simulink library "vmc"  (R2021b)
settings: Solver=VariableStepAuto  StartTime=0.0  StopTime=10.0  RelTol=1e-3
undefined symbols (not defined in the file or in its folder): AVMC_ACCDeltaTqIGain_X_kph, AVMC_ACCDeltaTqIGain_Y_mps2, AVMC_ACCDeltaTqPGain_X_kph, AVMC_ACCDeltaTqPGain_Y_kph, AVMC_ACCLongSteadyCtrl_X_kph, AVMC_AggressJerkPCT4AT_X_kph, AVMC_AggressJerkPCT_X_kph, AVMC_AggressLimitPCT4AT_X_kph, AVMC_AggressLimitPCT_X_kph, AVMC_CCLongSteadyCtrl_X_kph, AVMC_DISCDeltaTqIGain_X_kph, AVMC_DISCDeltaTqIGain_Y_mps2, AVMC_DISCDeltaTqPGain_X_kph, AVMC_DISCDeltaTqPGain_Y_kph, AVMC_DISCTrunAccJerk_X_s, AVMC_DISCTrunAccLimit_X_s, AVMC_ESCRegenOut_X_kph, AVMC_ESCRegenOut_Y_Deg, AVMC_ESCRegenOutEnSpd_X_Deg, AVMC_ISOAccLimit_X_mps, AVMC_ISODecLimit_X_mps, AVMC_ISOJerk_X_mps, AVMC_LatESCRegenOut_X_kph, AVMC_LatESCRegenOut_Y_Deg, AVMC_LongAccDeadZone_X_kph, AVMC_LongAccFiltTsforP2_X_Gps, AVMC_MCPresBaseTq_X_bar, AVMC_MSALongSteadyCtrl_X_kph, AVMC_MSAPedalOvrd2_X_kph, AVMC_MSAPedalOvrd_X_kph, AVMC_MSASpdBand_X_kph, AVMC_MSATqDownEndTq_X_kph, AVMC_MSATqDownTime_X_kph, AVMC_RDCDetectTime_X_kph, AVMC_RDCDetectTime_Y_pct, AVMC_RDCEnSlideRate_X_Deg, AVMC_RearWhlTqRatio_X_Nm, AVMC_RearWhlTqRatio_Y_gps, AVMC_RearWhlTqSlipGain_X_rat, AVMC_RearWhlTqSlipGain_Y_kph, AVMC_SoftJerkPCT_X_kph, AVMC_SoftLimitPCT_X_kph, AVMC_StESCYaw_X_kph, AVMC_StESCYaw_Y_Deg, AVMC_StESCYawCom_X_kph, AVMC_StESCYawCom_Y_Gps, AVMC_TMSpdBaseTq_X_rpm, AVMC_VehHoldBDecMap_X_kph, AVMC_VehHoldDecCtrlTime_X_kph, AVMC_VehHoldMCPPass_X_deg, C_TASK_10MS_S, C_TASK_5MS_S, DEG2RAD, Discrete, ENUM_ACCAVAIL_AVAILABLE, ENUM_ACCCTRLALLOW_ALLOW, ENUM_ADASACCSTA_ACTIVE, ENUM_ADASACCSTA_OVERRIDE, ENUM_ADASACCSTA_SHUTOFF, ENUM_ADASAEBREQ_NOREQUEST ... (+361)
libraries: hcu_lib x63, simulink x60, simulink_extras x3, ctrlSharedLib x3, $bdroot x2
(part 3 of 15)

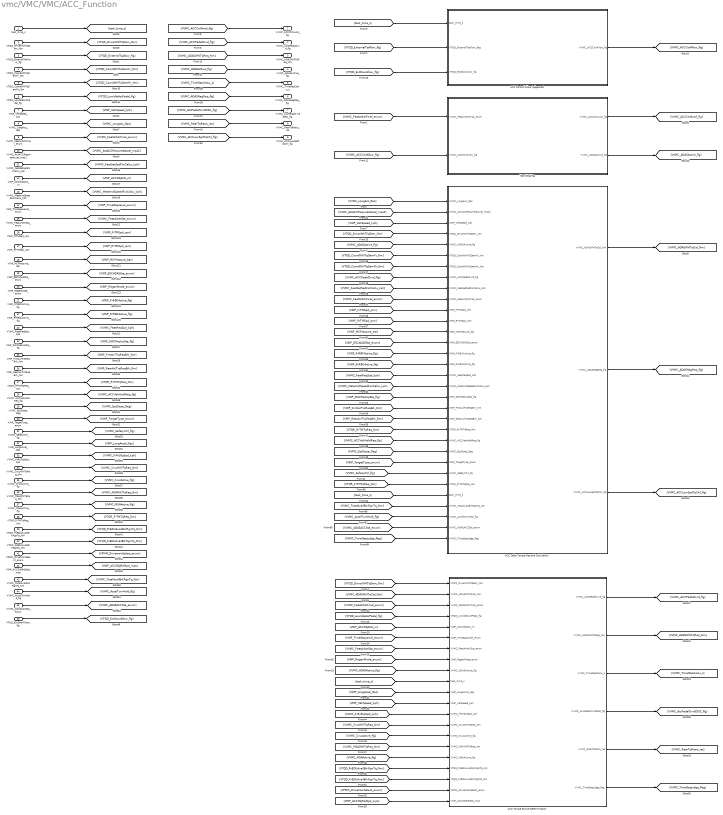
== system vmc/VMC/VMC/ACC_Function ==
  task_time_s : Inport
  VTQD_DriverWhlTqDem_Nm : Inport  Port=2
  VTQD_ExternalTqAllow_flg : Inport  Port=3
  VTQD_CoordWhlTqDemFr_Nm : Inport  Port=4
  VTQD_CoordWhlTqDemRr_Nm : Inport  Port=5
  VTQD_LowIdleAccPedal_flg : Inport  Port=6
  VINP_VehSpeed_kph : Inport  Port=7
  VVMC_LongAcc_Gps : Inport  Port=8
  VVMC_FeatArbitrFinal_enum : Inport  Port=9
  VVMC_ActACCRequiredAccel_mps2 : Inport  Port=10
  VVMC_FeatSetSpdForCalcu_kph : Inport  Port=11
  VINP_ACCObjDist_m : Inport  Port=12
  VVMC_MeterIndSpeedForCalcu_kph : Inport  Port=13
  VINP_TimeGapLevel_enum : Inport  Port=14
  VVMC_FeatArbitrSta_enum : Inport  Port=15
  VINP_FrTMSpd_rpm : Inport  Port=16
  VINP_RrTMSpd_rpm : Inport  Port=17
  VINP_MCPressure_bar : Inport  Port=18
  VINP_ESCADASSta_enum : Inport  Port=19
  VINP_RegenMode_enum : Inport  Port=20
  VINP_FrRBCActive_flg : Inport  Port=21
  VINP_RrRBCActive_flg : Inport  Port=22
  VVMC_FeatReqSpd_kph : Inport  Port=23
  VINP_SWCResUpSta_flg : Inport  Port=24
  VINP_FrntAxlTrqReqBrk_Nm : Inport  Port=25
  VINP_RearAxlTrqReqBrk_Nm : Inport  Port=26
  VTQR_RrTMTqReq_Nm : Inport  Port=27
  VVMC_ACCVehHoldReq_flg : Inport  Port=28
  VVMC_EstSlope_Deg : Inport  Port=29
  VINP_TargetType_enum : Inport  Port=30
  VVMC_SafetyCtrl_flg : Inport  Port=31
  VINP_LongAccel_Gps : Inport  Port=32
  VVMC_FrRrSlipSpd_kph : Inport  Port=33
  VVMC_CruzWhlTqReq_Nm : Inport  Port=34
  VVMC_CruzActive_flg : Inport  Port=35
  VVMC_MSAWhlTqReq_Nm : Inport  Port=36
  VVMC_MSAActive_flg : Inport  Port=37
  VTQR_FrTMTqReq_Nm : Inport  Port=38
  VTQD_RrEDUAvailBrkRgnTq_Nm : Inport  Port=39
  VTQD_FrEDUAvailBrkRgnTq_Nm : Inport  Port=40
  VPMM_DrivetrainSelect_enum : Inport  Port=41
  VINP_ACCObjRelSpd_mps : Inport  Port=42
  VVMC_TotalAvailBrkRgnTq_Nm : Inport  Port=43
  VVMC_AccelTurnHold_flg : Inport  Port=44
  VVMC_ADASACCSta_enum : Inport  Port=45
  VTQD_ExtDoorAllow_flg : Inport  Port=46
  ACC Control Allow Judgement : Subsystem
  ACC Delta Torque Map and Calculation : Subsystem
  ACC Torque Source Determination : Subsystem
  Hand Shaking : Subsystem
  VVMC_ACCCtrlAvail_flg : Outport
  VVMC_ACCPedalOvrd_flg : Outport  Port=2
  VVMC_ADASWhlTqReq_Nm : Outport  Port=3
  VVMC_ADASActive_flg : Outport  Port=4
  VVMC_TimeGapCalcu_s : Outport  Port=5
  VVMC_ADASNegReq_flg : Outport  Port=6
  VVMC_AccPedalOvrdDISC_flg : Outport  Port=7
  VVMC_RearTqRatio_rat : Outport  Port=8
  VVMC_ACCLowSpdTqCtrl_flg : Outport  Port=9
  wires:
  [VVMC_FeatReqSpd_kph] -> ACC Delta Torque Map and Calculation/17(VVMC_FeatReqSpd_kph)
  VVMC_FeatReqSpd_kph/1 -> [VVMC_FeatReqSpd_kph]
  [VVMC_ADASActive_flg] -> ACC Torque Source Determination/9(VVMC_ADASActive_flg)
  [VINP_RrRBCActive_flg] -> ACC Delta Torque Map and Calculation/16(VINP_RrRBCActive_flg)
  [VINP_FrRBCActive_flg] -> ACC Delta Torque Map and Calculation/15(VINP_FrRBCActive_flg)
  [VINP_ESCADASSta_enum] -> ACC Delta Torque Map and Calculation/14(VINP_ESCADASSta_enum)
  [VINP_MCPressure_bar] -> ACC Delta Torque Map and Calculation/13(VINP_MCPressure_bar)
  [VINP_RrTMSpd_rpm] -> ACC Delta Torque Map and Calculation/12(VINP_RrTMSpd_rpm)
  [VINP_FrTMSpd_rpm] -> ACC Delta Torque Map and Calculation/11(VINP_FrTMSpd_rpm)
  [VINP_RegenMode_enum] -> ACC Torque Source Determination/8(VINP_RegenMode_enum)
  VINP_FrTMSpd_rpm/1 -> [VINP_FrTMSpd_rpm]
  VINP_RrTMSpd_rpm/1 -> [VINP_RrTMSpd_rpm]
  VINP_MCPressure_bar/1 -> [VINP_MCPressure_bar]
  VINP_ESCADASSta_enum/1 -> [VINP_ESCADASSta_enum]
  VINP_RegenMode_enum/1 -> [VINP_RegenMode_enum]
  VINP_RrRBCActive_flg/1 -> [VINP_RrRBCActive_flg]
  VINP_FrRBCActive_flg/1 -> [VINP_FrRBCActive_flg]
  [VVMC_FeatArbitrFinal_enum] -> ACC Delta Torque Map and Calculation/10(VVMC_FeatArbitrFinal_enum)
  [VTQD_ExternalTqAllow_flg] -> ACC Control Allow Judgement/2(VTQD_ExternalTqAllow_flag)
  ACC Control Allow Judgement/1(VVMC_ACCCtrlAllow_flg) -> [VVMC_ACCCtrlAllow_flg]
  [task_time_s] -> ACC Control Allow Judgement/1(task_time_s)
  [VVMC_TimeGapCalcu_s] -> VVMC_TimeGapCalcu_s/1
  ACC Torque Source Determination/3(VVMC_TimeGapCalcu_s) -> [VVMC_TimeGapCalcu_s]
  [VVMC_FeatArbitrSta_enum] -> ACC Torque Source Determination/7(VVMC_FeatArbitrSta_enum)
  VVMC_FeatArbitrSta_enum/1 -> [VVMC_FeatArbitrSta_enum]
  [VINP_TimeGapLevel_enum] -> ACC Torque Source Determination/6(VINP_TimeGapLevel_enum)
  [VINP_ACCObjDist_m] -> ACC Torque Source Determination/5(VINP_ACCObjDist_m)
  VINP_TimeGapLevel_enum/1 -> [VINP_TimeGapLevel_enum]
  VINP_ACCObjDist_m/1 -> [VINP_ACCObjDist_m]
  VVMC_MeterIndSpeedForCalcu_kph/1 -> [VVMC_MeterIndSpeedForCalcu_kph]
  [VVMC_ACCPedalOvrd_flg] -> VVMC_ACCPedalOvrd_flg/1
  Hand Shaking/1(VVMC_ACCCtrlAvail_flg) -> [VVMC_ACCCtrlAvail_flg]
  VVMC_LongAcc_Gps/1 -> [VVMC_LongAcc_Gps]
  VVMC_FeatArbitrFinal_enum/1 -> [VVMC_FeatArbitrFinal_enum]
  VVMC_ActACCRequiredAccel_mps2/1 -> [VVMC_ActACCRequiredAccel_mps2]
  [VVMC_ACCCtrlAvail_flg] -> VVMC_ACCCtrlAvail_flg/1
  VTQD_ExternalTqAllow_flg/1 -> [VTQD_ExternalTqAllow_flg]
  VINP_VehSpeed_kph/1 -> [VINP_VehSpeed_kph]
  VTQD_DriverWhlTqDem_Nm/1 -> [VTQD_DriverWhlTqDem_Nm]
  [VVMC_LongAcc_Gps] -> ACC Delta Torque Map and Calculation/1(VVMC_LongAcc_Gps)
  [VVMC_ActACCRequiredAccel_mps2] -> ACC Delta Torque Map and Calculation/2(VVMC_ActACCRequiredAccel_mps2)
  [VINP_VehSpeed_kph] -> ACC Delta Torque Map and Calculation/3(VINP_VehSpeed_kph)
  [VTQD_DriverWhlTqDem_Nm] -> ACC Delta Torque Map and Calculation/4(VTQD_DriverWhlTqDem_Nm)
  ACC Delta Torque Map and Calculation/1(VVMC_ADASWhlTqCal_Nm) -> [VVMC_ADASWhlTqCal_Nm]
  [VTQD_DriverWhlTqDem_Nm] -> ACC Torque Source Determination/1(VTQD_DriverWhlTqDem_Nm)
  [VVMC_ADASWhlTqCal_Nm] -> ACC Torque Source Determination/2(VVMC_ADASWhlTqCal_Nm)
  ACC Torque Source Determination/1(VVMC_ACCPedalOvrd_flg) -> [VVMC_ACCPedalOvrd_flg]
  [VVMC_FeatArbitrFinal_enum] -> Hand Shaking/1(VVMC_FeatArbitrFinal_enum)
  Hand Shaking/2(VVMC_ADASActive_flg) -> [VVMC_ADASActive_flg]
  [VVMC_ADASActive_flg] -> ACC Delta Torque Map and Calculation/5(VVMC_ADASActive_flg)
  task_time_s/1 -> [task_time_s]
  [VVMC_ACCCtrlAllow_flg] -> Hand Shaking/2(VVMC_ACCCtrlAllow_flg)
  [VVMC_ADASActive_flg] -> VVMC_ADASActive_flg/1
  ACC Torque Source Determination/2(VVMC_ADASWhlTqReq_Nm) -> [VVMC_ADASWhlTqReq_Nm]
  [VVMC_ADASWhlTqReq_Nm] -> VVMC_ADASWhlTqReq_Nm/1
  [VTQD_CoordWhlTqDemFr_Nm] -> ACC Delta Torque Map and Calculation/6(VTQD_CoordWhlTqDemFr_Nm)
  [VTQD_CoordWhlTqDemRr_Nm] -> ACC Delta Torque Map and Calculation/7(VTQD_CoordWhlTqDemRr_Nm)
  VTQD_CoordWhlTqDemRr_Nm/1 -> [VTQD_CoordWhlTqDemRr_Nm]
  VTQD_CoordWhlTqDemFr_Nm/1 -> [VTQD_CoordWhlTqDemFr_Nm]
  [VVMC_ACCPedalOvrd_flg] -> ACC Delta Torque Map and Calculation/8(VVMC_ACCPedalOvrd_flg)
  [VVMC_FeatArbitrFinal_enum] -> ACC Torque Source Determination/3(VVMC_FeatArbitrFinal_enum)
  VTQD_LowIdleAccPedal_flg/1 -> [VTQD_LowIdleAccPedal_flg]
  [VTQD_LowIdleAccPedal_flg] -> ACC Torque Source Determination/4(VTQD_LowIdleAccPedal_flg)
  VVMC_FeatSetSpdForCalcu_kph/1 -> [VVMC_FeatSetSpdForCalcu_kph]
  [VVMC_FeatSetSpdForCalcu_kph] -> ACC Delta Torque Map and Calculation/9(VVMC_FeatSetSpdForCalcu_kph)
  VINP_SWCResUpSta_flg/1 -> [VINP_SWCResUpSta_flg]
  VINP_FrntAxlTrqReqBrk_Nm/1 -> [VINP_FrntAxlTrqReqBrk_Nm]
  VINP_RearAxlTrqReqBrk_Nm/1 -> [VINP_RearAxlTrqReqBrk_Nm]
  [VVMC_MeterIndSpeedForCalcu_kph] -> ACC Delta Torque Map and Calculation/18(VVMC_MeterIndSpeedForCalcu_kph)
  [VINP_SWCResUpSta_flg] -> ACC Delta Torque Map and Calculation/19(VINP_SWCResUpSta_flg)
  [VINP_FrntAxlTrqReqBrk_Nm] -> ACC Delta Torque Map and Calculation/20(VINP_FrntAxlTrqReqBrk_Nm)
  [VINP_RearAxlTrqReqBrk_Nm] -> ACC Delta Torque Map and Calculation/21(VINP_RearAxlTrqReqBrk_Nm)
  ACC Delta Torque Map and Calculation/2(VVMC_ADASNegReq_flg) -> [VVMC_ADASNegReq_flg]
  [VVMC_ADASNegReq_flg] -> VVMC_ADASNegReq_flg/1
  VTQR_RrTMTqReq_Nm/1 -> [VTQR_RrTMTqReq_Nm]
  [VTQR_RrTMTqReq_Nm] -> ACC Delta Torque Map and Calculation/22(VTQR_RrTMTqReq_Nm)
  ACC Torque Source Determination/4(VVMC_AccPedalOvrdDISC_flg) -> [VVMC_AccPedalOvrdDISC_flg]
  [VVMC_AccPedalOvrdDISC_flg] -> VVMC_AccPedalOvrdDISC_flg/1
  VVMC_ACCVehHoldReq_flg/1 -> [VVMC_ACCVehHoldReq_flg]
  [VVMC_ACCVehHoldReq_flg] -> ACC Delta Torque Map and Calculation/23(VVMC_ACCVehHoldReq_flg)
  VVMC_EstSlope_Deg/1 -> [VVMC_EstSlope_Deg]
  [VVMC_EstSlope_Deg] -> ACC Delta Torque Map and Calculation/24(VVMC_EstSlope_Deg)
  [VINP_TargetType_enum] -> ACC Delta Torque Map and Calculation/25(VINP_TargetType_enum)
  VINP_TargetType_enum/1 -> [VINP_TargetType_enum]
  [task_time_s] -> ACC Torque Source Determination/10(task_time_s)
  VVMC_SafetyCtrl_flg/1 -> [VVMC_SafetyCtrl_flg]
  [VVMC_SafetyCtrl_flg] -> ACC Delta Torque Map and Calculation/26(VVMC_SafetyCtrl_flg)
  [VINP_LongAccel_Gps] -> ACC Torque Source Determination/11(VINP_LongAccel_Gps)
  ACC Torque Source Determination/5(VVMC_RearTqRatio_rat) -> [VVMC_RearTqRatio_rat]
  [VVMC_RearTqRatio_rat] -> VVMC_RearTqRatio_rat/1
  VINP_LongAccel_Gps/1 -> [VINP_LongAccel_Gps]
  VVMC_FrRrSlipSpd_kph/1 -> [VVMC_FrRrSlipSpd_kph]
  [VINP_VehSpeed_kph] -> ACC Torque Source Determination/12(VINP_VehSpeed_kph)
  [VVMC_FrRrSlipSpd_kph] -> ACC Torque Source Determination/13(VVMC_FrRrSlipSpd_kph)
  VVMC_MSAActive_flg/1 -> [VVMC_MSAActive_flg]
  VVMC_MSAWhlTqReq_Nm/1 -> [VVMC_MSAWhlTqReq_Nm]
  VVMC_CruzActive_flg/1 -> [VVMC_CruzActive_flg]
  VVMC_CruzWhlTqReq_Nm/1 -> [VVMC_CruzWhlTqReq_Nm]
  [VVMC_CruzWhlTqReq_Nm] -> ACC Torque Source Determination/14(VVMC_CruzWhlTqReq_Nm)
  [VVMC_CruzActive_flg] -> ACC Torque Source Determination/15(VVMC_CruzActive_flg)
  [VVMC_MSAWhlTqReq_Nm] -> ACC Torque Source Determination/16(VVMC_MSAWhlTqReq_Nm)
  [VVMC_MSAActive_flg] -> ACC Torque Source Determination/17(VVMC_MSAActive_flg)
  [VTQR_FrTMTqReq_Nm] -> ACC Delta Torque Map and Calculation/27(VTQR_FrTMTqReq_Nm)
  VTQR_FrTMTqReq_Nm/1 -> [VTQR_FrTMTqReq_Nm]
  VTQD_RrEDUAvailBrkRgnTq_Nm/1 -> [VTQD_RrEDUAvailBrkRgnTq_Nm]
  VTQD_FrEDUAvailBrkRgnTq_Nm/1 -> [VTQD_FrEDUAvailBrkRgnTq_Nm]
  [VTQD_RrEDUAvailBrkRgnTq_Nm] -> ACC Torque Source Determination/18(VTQD_RrEDUAvailBrkRgnTq_Nm)
  [VTQD_FrEDUAvailBrkRgnTq_Nm] -> ACC Torque Source Determination/19(VTQD_FrEDUAvailBrkRgnTq_Nm)
  ACC Delta Torque Map and Calculation/3(VVMC_ACCLowSpdTqCtrl_flg) -> [VVMC_ACCLowSpdTqCtrl_flg]
  [VVMC_ACCLowSpdTqCtrl_flg] -> VVMC_ACCLowSpdTqCtrl_flg/1
  VPMM_DrivetrainSelect_enum/1 -> [VPMM_DrivetrainSelect_enum]
  [VPMM_DrivetrainSelect_enum] -> ACC Torque Source Determination/20(VPMM_DrivetrainSelect_enum)
  [task_time_s] -> ACC Delta Torque Map and Calculation/28(task_time_s)
  VINP_ACCObjRelSpd_mps/1 -> [VINP_ACCObjRelSpd_mps]
  [VINP_ACCObjRelSpd_mps] -> ACC Torque Source Determination/21(VINP_ACCObjRelSpd_mps)
  VVMC_TotalAvailBrkRgnTq_Nm/1 -> [VVMC_TotalAvailBrkRgnTq_Nm]
  [VVMC_TotalAvailBrkRgnTq_Nm] -> ACC Delta Torque Map and Calculation/29(VVMC_TotalAvailBrkRgnTq_Nm)
  VVMC_AccelTurnHold_flg/1 -> [VVMC_AccelTurnHold_flg]
  [VVMC_AccelTurnHold_flg] -> ACC Delta Torque Map and Calculation/30(VVMC_AccelTurnHold_flg)
  VVMC_ADASACCSta_enum/1 -> [VVMC_ADASACCSta_enum]
  [VVMC_ADASACCSta_enum] -> ACC Delta Torque Map and Calculation/31(VVMC_ADASACCSta_enum)
  ACC Torque Source Determination/6(VVMC_TimeGapJudge_flag) -> [VVMC_TimeGapJudge_flag]
  [VVMC_TimeGapJudge_flag] -> ACC Delta Torque Map and Calculation/32(VVMC_TimeGapJudge_flag)
  [VTQD_ExtDoorAllow_flg] -> ACC Control Allow Judgement/3(VTQD_ExtDoorAllow_flg)
  VTQD_ExtDoorAllow_flg/1 -> [VTQD_ExtDoorAllow_flg]

== system vmc/VMC/VMC/APS function ==
  VTQD_ExternalTqAllow_flg : Inport
  VTQD_ExtShiftAllow_flg : Inport  Port=2
  VTQD_ExtDoorAllow_flg : Inport  Port=3
  VTQD_GearActualPosn_enum : Inport  Port=4
  VINP_APSStaSys_enum : Inport  Port=5
  VINP_APSVMCReqA_flg : Inport  Port=6
  VINP_APSShiftPosnReq_enum : Inport  Port=7
  VINP_APSSpeedCMD_kph : Inport  Port=8
  task_time_s : Inport  Port=9
  VINP_SCPSystemMode_enum : Inport  Port=10
  VVMC_ADASActive_flg : Inport  Port=11
  BINP_APM_outputs : Inport  Port=12  OutDataTypeStr=Bus: BINP_APM_outputs
  VTQD_APSStaSys_enum : Inport  Port=13
  VTQD_APSDecReqA_flg : Inport  Port=14
  VTQD_APSDecReq_mps2 : Inport  Port=15
  VTQD_APSReq_enum : Inport  Port=16
  Command Determination : Subsystem
  Data Type Conversion : DataTypeConversion  OutDataTypeStr=uint8
  Hand Shake : Subsystem
  Signal Rounting : Subsystem
  VVMC_APSCtrlAvail_flg : Outport
  VVMC_APSActive_flg : Outport  Port=2
  VVMC_APSSpeedCMD_kph : Outport  Port=3
  VVMC_APSShiftPosnReq_enum : Outport  Port=4
  VVMC_APSStaSys_enum : Outport  Port=5
  VVMC_APSDecReqA_flg : Outport  Port=6
  VVMC_APSDecReq_mps2 : Outport  Port=7
  VVMC_APSReq_enum : Outport  Port=8
  wires:
  Command Determination/2(VVMC_APSShiftPosnReq_enum) -> VVMC_APSShiftPosnReq_enum/1
  Command Determination/1(VVMC_APSSpeedCMD_kph) -> VVMC_APSSpeedCMD_kph/1
  [VINP_APSSpeedCMD_kph] -> Command Determination/4(VINP_APSSpeedCMD_kph)
  [VINP_APSShiftPosnReq_enum] -> Command Determination/3(VINP_APSShiftPosnReq_enum)
  [VINP_APSStaSys_enum] -> Command Determination/2(VINP_APSStaSys_enum)
  [VVMC_APSActive_flg] -> Command Determination/1(VVMC_APSActive_flg)
  Hand Shake/1(VVMC_APSCtrlAvail_flg) -> VVMC_APSCtrlAvail_flg/1
  Hand Shake/2(VVMC_APSActive_flg) -> VVMC_APSActive_flg/1, [VVMC_APSActive_flg]
  [VTQD_ExtShiftAllow_flg] -> Hand Shake/3(VTQD_ExtShiftAllow_flg)
  [VTQD_ExternalTqAllow_flg] -> Hand Shake/2(VTQD_ExternalTqAllow_flg)
  [task_time_s] -> Hand Shake/1(task_time_s)
  task_time_s/1 -> [task_time_s]
  VINP_APSSpeedCMD_kph/1 -> [VINP_APSSpeedCMD_kph]
  VINP_APSShiftPosnReq_enum/1 -> [VINP_APSShiftPosnReq_enum]
  VINP_APSVMCReqA_flg/1 -> [VINP_APSVMCReqA_flg]
  VINP_APSStaSys_enum/1 -> [VINP_APSStaSys_enum]
  VVMC_ADASActive_flg/1 -> [VVMC_ADASActive_flg]
  [VVMC_APSActive_flg] -> Signal Rounting/2(VVMC_APSActive_flg)
  [VVMC_ADASActive_flg] -> Signal Rounting/3(VVMC_ADASActive_flg)
  Signal Rounting/1(VVMC_APSStaSys_enum) -> VVMC_APSStaSys_enum/1
  Signal Rounting/4(VVMC_APSReq_enum) -> VVMC_APSReq_enum/1
  Signal Rounting/3(VVMC_APSDecReq_mps2) -> VVMC_APSDecReq_mps2/1
  Signal Rounting/2(VVMC_APSDecReqA_flg) -> VVMC_APSDecReqA_flg/1
  VTQD_ExtDoorAllow_flg/1 -> [VTQD_ExtDoorAllow_flg]
  VTQD_ExternalTqAllow_flg/1 -> [VTQD_ExternalTqAllow_flg]
  VTQD_ExtShiftAllow_flg/1 -> [VTQD_ExtShiftAllow_flg]
  VINP_SCPSystemMode_enum/1 -> Data Type Conversion/1
  [VTQD_ExtDoorAllow_flg] -> Hand Shake/6(VTQD_ExtDoorAllow_flg)
  [BINP_APM_outputs] -> Signal Rounting/4(BINP_APM_outputs)
  [VINP_APSVMCReqA_flg] -> Hand Shake/4(VINP_APSVMCReqA_flg)
  [VINP_APSStaSys_enum] -> Hand Shake/5(VINP_APSStaSys_enum)
  BINP_APM_outputs/1 -> [BINP_APM_outputs]
  VTQD_GearActualPosn_enum/1 -> [VTQD_GearActualPosn_enum]
  [VINP_SCPSystemMode_enum] -> Signal Rounting/1(VINP_SCPSystemMode_enum)
  [VTQD_GearActualPosn_enum] -> Signal Rounting/5(VTQD_GearActualPosn_enum)
  Data Type Conversion/1 -> [VINP_SCPSystemMode_enum]
  VTQD_APSStaSys_enum/1 -> [VTQD_APSStaSys_enum]
  VTQD_APSDecReq_mps2/1 -> [VTQD_APSDecReq_mps2]
  VTQD_APSDecReqA_flg/1 -> [VTQD_APSDecReqA_flg]
  VTQD_APSReq_enum/1 -> [VTQD_APSReq_enum]
  [VTQD_APSStaSys_enum] -> Signal Rounting/6(VTQD_APSStaSys_enum)
  [VTQD_APSDecReqA_flg] -> Signal Rounting/7(VTQD_APSDecReqA_flg)
  [VTQD_APSDecReq_mps2] -> Signal Rounting/8(VTQD_APSDecReq_mps2)
  [VTQD_APSReq_enum] -> Signal Rounting/9(VTQD_APSReq_enum)

== system vmc/VMC/VMC/CruiseControlFunction ==
  VTQD_ExternalTqAllow_flg : Inport
  VTQD_DriverWhlTqDem_Nm : Inport  Port=2
  VTQD_LowIdleAccPedal_flg : Inport  Port=3
  <VINP_ZoneSpdCtrlMode_enum> : Inport  Port=4
  VINP_SWCResUpSta_flg : Inport  Port=5
  VINP_SWCSetdownSta_flg : Inport  Port=6
  VINP_SWCCANCELSta_flg : Inport  Port=7
  VINP_BrakeSWGPIO_flg : Inport  Port=8
  VINP_BrkSwSta_flg : Inport  Port=9
  VINP_VehSpeed_kph : Inport  Port=10
  VVMC_LongAcc_Gps : Inport  Port=11
  VVMC_FeatSetSpdForCalcu_kph : Inport  Port=12
  VVMC_FeatArbitrFinal_enum : Inport  Port=13
  VINP_ADASAEBSta_enum : Inport  Port=14
  VTQD_GearActualPosn_enum : Inport  Port=15
  VVMC_CalMeterSpeed_kph : Inport  Port=16
  VVMC_MeterIndSpeedForCalcu_kph : Inport  Port=17
  VVMC_SafetyCtrl_flg : Inport  Port=18
  VTQR_FrTMTqReq_Nm : Inport  Port=19
  VTQR_RrTMTqReq_Nm : Inport  Port=20
  VINP_RegenMode_enum : Inport  Port=21
  VVMC_ActACCRequiredAccel_mps2 : Inport  Port=22
  task_time_s : Inport  Port=23
  VVMC_TotalAvailBrkRgnTq_Nm : Inport  Port=24
  CCActiveDetermination : Subsystem
  CCDemandTorqueCalculation : Subsystem
  CCTorqueSourceDetermination : Subsystem
  Data Type Conversion : DataTypeConversion  OutDataTypeStr=single
  VVMC_CCCtrlSta_enum : Outport
  VVMC_CCSpdWar_flg : Outport  Port=2
  VVMC_CruzWhlTqReq_Nm : Outport  Port=3
  VVMC_CruzActive_flg : Outport  Port=4
  VVMC_CCPedalOvrd_flg : Outport  Port=5
  wires:
  [VVMC_CCPedalOvrd_flg] -> VVMC_CCPedalOvrd_flg/1
  [VVMC_CCPedalOvrd_flg] -> CCActiveDetermination/12(VVMC_CCPedalOvrd_flg)
  [VINP_ADASAEBSta_enum] -> CCActiveDetermination/11(VINP_ADASAEBSta_enum)
  VINP_ADASAEBSta_enum/1 -> [VINP_ADASAEBSta_enum]
  [VINP_ZoneSpdCtrlMode_enum] -> CCActiveDetermination/1(VINP_ZoneSpdCtrlMode_enum)
  <VINP_ZoneSpdCtrlMode_enum>/1 -> [VINP_ZoneSpdCtrlMode_enum]
  [VVMC_FeatArbitrFinal_enum] -> CCActiveDetermination/2(VVMC_FeatArbitrFinal_enum)
  [VTQD_ExternalTqAllow_flg] -> CCActiveDetermination/3(VTQD_ExternalTqAllow_flg)
  [VINP_SWCSetdownSta_flg] -> CCActiveDetermination/4(VINP_SWCSetdownSta_flg)
  [VINP_SWCResUpSta_flg] -> CCActiveDetermination/5(VINP_SWCResUpSta_flg)
  [VVMC_FeatSetSpdForCalcu_kph] -> CCActiveDetermination/7(VVMC_FeatSetSpdForCalcu_kph)
  [VINP_BrakeSWGPIO_flg] -> CCActiveDetermination/8(VINP_BrakeSWGPIO_flg)
  [VINP_SWCCANCELSta_flg] -> CCActiveDetermination/9(VINP_SWCCANCELSta_flg)
  [VINP_BrkSwSta_flg] -> CCActiveDetermination/10(VINP_BrkSwSta_flg)
  [VVMC_FeatSetSpdForCalcu_kph] -> CCDemandTorqueCalculation/1(VVMC_FeatSetSpdForCalcu_kph)
  [VINP_VehSpeed_kph] -> CCDemandTorqueCalculation/2(VINP_VehSpeed_kph)
  [VVMC_CruzActive_flg] -> CCDemandTorqueCalculation/3(VVMC_CruzActive_flg)
  [VTQD_DriverWhlTqDem_Nm] -> CCDemandTorqueCalculation/4(VTQD_DriverWhlTqDem_Nm)
  [VTQD_DriverWhlTqDem_Nm] -> CCTorqueSourceDetermination/1(VTQD_DriverWhlTqDem_Nm)
  [VVMC_CruzWhlTqCal_Nm] -> CCTorqueSourceDetermination/2(VVMC_CruzWhlTqCal_Nm)
  CCActiveDetermination/1(VVMC_CCCtrlSta_enum) -> [VVMC_CCCtrlSta_enum]
  CCActiveDetermination/2(VVMC_CCSpdWar_flg) -> [VVMC_CCSpdWar_flg]
  CCActiveDetermination/3(VVMC_CruzActive_flg) -> [VVMC_CruzActive_flg]
  CCDemandTorqueCalculation/1(VVMC_CruzWhlTqCal_Nm) -> [VVMC_CruzWhlTqCal_Nm]
  CCTorqueSourceDetermination/1(VVMC_CruzWhlTqReq_Nm) -> [VVMC_CruzWhlTqReq_Nm]  "VVMC_CruzWhlTqReq_Nm"
  VTQD_ExternalTqAllow_flg/1 -> [VTQD_ExternalTqAllow_flg]
  VTQD_DriverWhlTqDem_Nm/1 -> [VTQD_DriverWhlTqDem_Nm]
  VINP_SWCResUpSta_flg/1 -> [VINP_SWCResUpSta_flg]
  VINP_SWCSetdownSta_flg/1 -> [VINP_SWCSetdownSta_flg]
  VINP_SWCCANCELSta_flg/1 -> [VINP_SWCCANCELSta_flg]
  VINP_BrakeSWGPIO_flg/1 -> [VINP_BrakeSWGPIO_flg]
  VVMC_FeatSetSpdForCalcu_kph/1 -> Data Type Conversion/1
  VINP_BrkSwSta_flg/1 -> [VINP_BrkSwSta_flg]
  VVMC_FeatArbitrFinal_enum/1 -> [VVMC_FeatArbitrFinal_enum]
  VINP_VehSpeed_kph/1 -> [VINP_VehSpeed_kph]
  [VVMC_CCCtrlSta_enum] -> VVMC_CCCtrlSta_enum/1
  [VVMC_CCSpdWar_flg] -> VVMC_CCSpdWar_flg/1
  [VVMC_CruzWhlTqReq_Nm] -> VVMC_CruzWhlTqReq_Nm/1
  Data Type Conversion/1 -> [VVMC_FeatSetSpdForCalcu_kph]  "VVMC_FeatSetSpdForCalcu_kph"
  [VVMC_CruzActive_flg] -> VVMC_CruzActive_flg/1
  VVMC_LongAcc_Gps/1 -> [VVMC_LongAcc_Gps]
  [VVMC_LongAcc_Gps] -> CCDemandTorqueCalculation/5(VVMC_LongAcc_Gps)
  [VINP_VehSpeed_kph] -> CCActiveDetermination/6(VINP_VehSpeed_kph)
  VTQD_LowIdleAccPedal_flg/1 -> [VTQD_LowIdleAccPedal_flg]
  [VTQD_LowIdleAccPedal_flg] -> CCTorqueSourceDetermination/3(VTQD_LowIdleAccPedal_flg)
  CCTorqueSourceDetermination/2(VVMC_CCPedalOvrd_flg) -> [VVMC_CCPedalOvrd_flg]  "VVMC_CCPedalOvrd_flg"
  [VVMC_CCPedalOvrd_flg] -> CCDemandTorqueCalculation/6(VVMC_CCPedalOvrd_flg)
  VTQD_GearActualPosn_enum/1 -> [VTQD_GearActualPosn_enum]
  [VTQD_GearActualPosn_enum] -> CCActiveDetermination/13(VTQD_GearActualPosn_enum)
  VVMC_CalMeterSpeed_kph/1 -> [VVMC_CalMeterSpeed_kph]
  [VVMC_CalMeterSpeed_kph] -> CCDemandTorqueCalculation/7(VVMC_CalMeterSpeed_kph)
  [VVMC_FeatArbitrFinal_enum] -> CCDemandTorqueCalculation/8(VVMC_FeatArbitrFinal_enum)
  [VVMC_MeterIndSpeedForCalcu_kph] -> CCDemandTorqueCalculation/10(VVMC_MeterIndSpeedForCalcu_kph)
  VVMC_MeterIndSpeedForCalcu_kph/1 -> [VVMC_MeterIndSpeedForCalcu_kph]
  [VVMC_SafetyCtrl_flg] -> CCDemandTorqueCalculation/11(VVMC_SafetyCtrl_flg)
  VVMC_SafetyCtrl_flg/1 -> [VVMC_SafetyCtrl_flg]
  [VTQR_FrTMTqReq_Nm] -> CCDemandTorqueCalculation/12(VTQR_FrTMTqReq_Nm)
  [VTQR_RrTMTqReq_Nm] -> CCDemandTorqueCalculation/13(VTQR_RrTMTqReq_Nm)
  VTQR_FrTMTqReq_Nm/1 -> [VTQR_FrTMTqReq_Nm]
  VTQR_RrTMTqReq_Nm/1 -> [VTQR_RrTMTqReq_Nm]
  [VINP_RegenMode_enum] -> CCTorqueSourceDetermination/4(VINP_RegenMode_enum)
  [VVMC_FeatArbitrFinal_enum] -> CCTorqueSourceDetermination/5(VVMC_FeatArbitrFinal_enum)
  VINP_RegenMode_enum/1 -> [VINP_RegenMode_enum]
  [task_time_s] -> CCTorqueSourceDetermination/6(task_time_s)
  VVMC_ActACCRequiredAccel_mps2/1 -> [VVMC_ActACCRequiredAccel_mps2]
  task_time_s/1 -> [task_time_s]
  [VVMC_ActACCRequiredAccel_mps2] -> CCDemandTorqueCalculation/9(VVMC_ActACCRequiredAccel_mps2)
  VVMC_TotalAvailBrkRgnTq_Nm/1 -> [VVMC_TotalAvailBrkRgnTq_Nm]
  [VVMC_TotalAvailBrkRgnTq_Nm] -> CCDemandTorqueCalculation/14(VVMC_TotalAvailBrkRgnTq_Nm)

== system vmc/VMC/VMC/FeatureSetSpeed ==
  APP_SpdLimit_flg : Inport
  VINP_ZoneSpdCtrlSta_flg : Inport  Port=2
  APP_SpdLimit : Inport  Port=3
  VINP_SetSpd_kph : Inport  Port=4
  VINP_Distanceunit_flg : Inport  Port=5
  Cast To Single : DataTypeConversion  OutDataTypeStr=single
  Cast To Single1 : DataTypeConversion  OutDataTypeStr=single
  Constant : Constant  Value=ENUM_SCPCRLSTA_ON
  Constant1 : Constant  Value=ENUM_APPSPDLIMIT_ON
  Constant2 : Constant  Value=ZERO_FLOAT
  Constant4 : Constant  Value=MPH2KPH
  Constant5 : Constant  Value=KVMC_APPSpdLimit_flg_ovrdflg
  Constant6 : Constant  Value=KVMC_APPSpdLimit_flg_ovrdval
  Constant7 : Constant  Value=KVMC_APPSpdLimit_ovrdflg
  Constant8 : Constant  Value=KVMC_APPSpdLimit_ovrdval
  Divide1 : Product  Inputs=**
  Round1 : Rounding  Operator=ceil
  SpeedDetermination : Stateflow chart  TreatAsAtomicUnit=on
  Switch : Switch  Criteria=u2 ~= 0
  Switch1 : Switch  Criteria=u2 ~= 0
  u2 > 0 (2) : Switch  Criteria=u2 > Threshold
  VVMC_FeatSetSpdFinal_raw32 : Outport
  VVMC_FeatSetSpdForCalcu_kph : Outport  Port=2
  wires:
  [VINP_SetSpd_kph] -> SpeedDetermination/4(VINP_SetSpd_kph)
  Constant2/1 -> SpeedDetermination/7(ZERO_FLOAT)
  Constant6/1 -> Switch/1
  Constant1/1 -> SpeedDetermination/6(ENUM_APPSPDLIMIT_ON)
  Constant5/1 -> Switch/2
  [APP_SpdLimit_flg] -> Switch/3
  SpeedDetermination/1(VVMC_FeatSetSpdFinal_raw32) -> Cast To Single/1
  Constant/1 -> SpeedDetermination/5(ENUM_SCPCRLSTA_ON)
  Switch1/1 -> [VVMC_APPSpdLimit_kph]  "VVMC_APPSpdLimit_kph"
  Constant8/1 -> Switch1/1
  [APP_SpdLimit] -> Switch1/3
  [VINP_ZoneSpdCtrlSta_flg] -> SpeedDetermination/2(VINP_ZoneSpdCtrlSta_flg)
  Constant7/1 -> Switch1/2
  [VVMC_APPSpdLimit_flg] -> SpeedDetermination/1(VVMC_APPSpdLimit_flg)
  Switch/1 -> [VVMC_APPSpdLimit_flg]  "VVMC_APPSpdLimit_flg"
  Cast To Single/1 -> [VVMC_FeatSetSpdFinal_raw32]  "VVMC_FeatSetSpdFinal_raw32"
  [VVMC_APPSpdLimit_kph] -> SpeedDetermination/3(VVMC_APPSpdLimit_kph)
  APP_SpdLimit_flg/1 -> [APP_SpdLimit_flg]
  VINP_ZoneSpdCtrlSta_flg/1 -> [VINP_ZoneSpdCtrlSta_flg]
  APP_SpdLimit/1 -> [APP_SpdLimit]
  VINP_SetSpd_kph/1 -> [VINP_SetSpd_kph]
  [VVMC_FeatSetSpdFinal_raw32] -> VVMC_FeatSetSpdFinal_raw32/1
  [VVMC_FeatSetSpdFinal_raw32] -> Divide1/1, u2 > 0 (2)/3
  u2 > 0 (2)/1 -> Cast To Single1/1
  Constant4/1 -> Divide1/2
  Divide1/1 -> u2 > 0 (2)/1
  [VINP_Distanceunit_flg] -> u2 > 0 (2)/2
  Round1/1 -> [VVMC_FeatSetSpdForCalcu_kph]  "VVMC_FeatSetSpdForCalcu_kph"
  Cast To Single1/1 -> Round1/1
  [VVMC_FeatSetSpdForCalcu_kph] -> VVMC_FeatSetSpdForCalcu_kph/1
  VINP_Distanceunit_flg/1 -> [VINP_Distanceunit_flg]

== system vmc/VMC/VMC/IMU ==
  VINP_MemOffsetGyroX_raw16 : Inport
  VINP_MemOffsetGyroY_raw16 : Inport  Port=2
  VINP_MemOffsetGyroZ_raw16 : Inport  Port=3
  VINP_MemOffsetAccX_raw16 : Inport  Port=4
  VINP_MemOffsetAccY_raw16 : Inport  Port=5
  VINP_MemOffsetAccZ_raw16 : Inport  Port=6
  VINP_SensingGyroX_raw16 : Inport  Port=7
  VINP_SensingGyroY_raw16 : Inport  Port=8
  VINP_SensingGyroZ_raw16 : Inport  Port=9
  VINP_SensingAccX_raw16 : Inport  Port=10
  VINP_SensingAccY_raw16 : Inport  Port=11
  VINP_SensingAccZ_raw16 : Inport  Port=12
  task_time_s : Inport  Port=13
  Constant : Constant  Value=KVMC_IMUEnaCmd_flg
  IMU memorized offset result : Subsystem
  "IMU sensing result " : Subsystem
  VVMC_IMUEnaCmd_flg : Outport
  wires:
  VINP_MemOffsetGyroX_raw16/1 -> [VINP_MemOffsetGyroX_raw16]
  VINP_MemOffsetGyroY_raw16/1 -> [VINP_MemOffsetGyroY_raw16]
  VINP_MemOffsetGyroZ_raw16/1 -> [VINP_MemOffsetGyroZ_raw16]
  VINP_MemOffsetAccX_raw16/1 -> [VINP_MemOffsetAccX_raw16]
  VINP_MemOffsetAccY_raw16/1 -> [VINP_MemOffsetAccY_raw16]
  VINP_MemOffsetAccZ_raw16/1 -> [VINP_MemOffsetAccZ_raw16]
  VINP_SensingGyroX_raw16/1 -> [VINP_SensingGyroX_raw16]
  VINP_SensingGyroY_raw16/1 -> [VINP_SensingGyroY_raw16]
  VINP_SensingGyroZ_raw16/1 -> [VINP_SensingGyroZ_raw16]
  VINP_SensingAccX_raw16/1 -> [VINP_SensingAccX_raw16]
  VINP_SensingAccY_raw16/1 -> [VINP_SensingAccY_raw16]
  VINP_SensingAccZ_raw16/1 -> [VINP_SensingAccZ_raw16]
  [VINP_MemOffsetGyroX_raw16] -> IMU memorized offset result/1(VINP_MemOffsetGyroX_raw16)
  [VINP_MemOffsetGyroY_raw16] -> IMU memorized offset result/2(VINP_MemOffsetGyroY_raw16)
  [VINP_MemOffsetGyroZ_raw16] -> IMU memorized offset result/3(VINP_MemOffsetGyroZ_raw16)
  [VINP_MemOffsetAccX_raw16] -> IMU memorized offset result/4(VINP_MemOffsetAccX_raw16)
  [VINP_MemOffsetAccY_raw16] -> IMU memorized offset result/5(VINP_MemOffsetAccY_raw16)
  [VINP_MemOffsetAccZ_raw16] -> IMU memorized offset result/6(VINP_MemOffsetAccZ_raw16)
  IMU memorized offset result/6(VVMC_MemOffsetAccZ_G) -> [VVMC_MemOffsetAccZ_G]
  IMU memorized offset result/5(VVMC_MemOffsetAccY_G) -> [VVMC_MemOffsetAccY_G]
  IMU memorized offset result/4(VVMC_MemOffsetAccX_G) -> [VVMC_MemOffsetAccX_G]
  IMU memorized offset result/3(VVMC_MemOffsetGyroZ_Dps) -> [VVMC_MemOffsetGyroZ_Dps]
  IMU memorized offset result/2(VVMC_MemOffsetGyroY_Dps) -> [VVMC_MemOffsetGyroY_Dps]
  IMU memorized offset result/1(VVMC_MemOffsetGyroX_Dps) -> [VVMC_MemOffsetGyroX_Dps]
  [VVMC_MemOffsetGyroY_Dps] -> "IMU sensing result "/8(VVMC_MemOffsetGyroY_Dps)
  [VVMC_MemOffsetAccX_G] -> "IMU sensing result "/10(VVMC_MemOffsetAccX_G)
  [VVMC_MemOffsetGyroZ_Dps] -> "IMU sensing result "/9(VVMC_MemOffsetGyroZ_Dps)
  [VVMC_MemOffsetAccY_G] -> "IMU sensing result "/11(VVMC_MemOffsetAccY_G)
  [VVMC_MemOffsetGyroX_Dps] -> "IMU sensing result "/7(VVMC_MemOffsetGyroX_Dps)
  [VVMC_MemOffsetAccZ_G] -> "IMU sensing result "/12(VVMC_MemOffsetAccZ_G)
  [VINP_SensingGyroX_raw16] -> "IMU sensing result "/1(VINP_SensingGyroX_raw16)
  [VINP_SensingAccZ_raw16] -> "IMU sensing result "/6(VINP_SensingAccZ_raw16)
  [VINP_SensingAccY_raw16] -> "IMU sensing result "/5(VINP_SensingAccY_raw16)
  [VINP_SensingAccX_raw16] -> "IMU sensing result "/4(VINP_SensingAccX_raw16)
  [VINP_SensingGyroZ_raw16] -> "IMU sensing result "/3(VINP_SensingGyroZ_raw16)
  [VINP_SensingGyroY_raw16] -> "IMU sensing result "/2(VINP_SensingGyroY_raw16)
  Constant/1 -> [VVMC_IMUEnaCmd_flg]  "VVMC_IMUEnaCmd_flg"
  [VVMC_IMUEnaCmd_flg] -> VVMC_IMUEnaCmd_flg/1
  task_time_s/1 -> [task_time_s]
  [task_time_s] -> "IMU sensing result "/13(task_time_s)

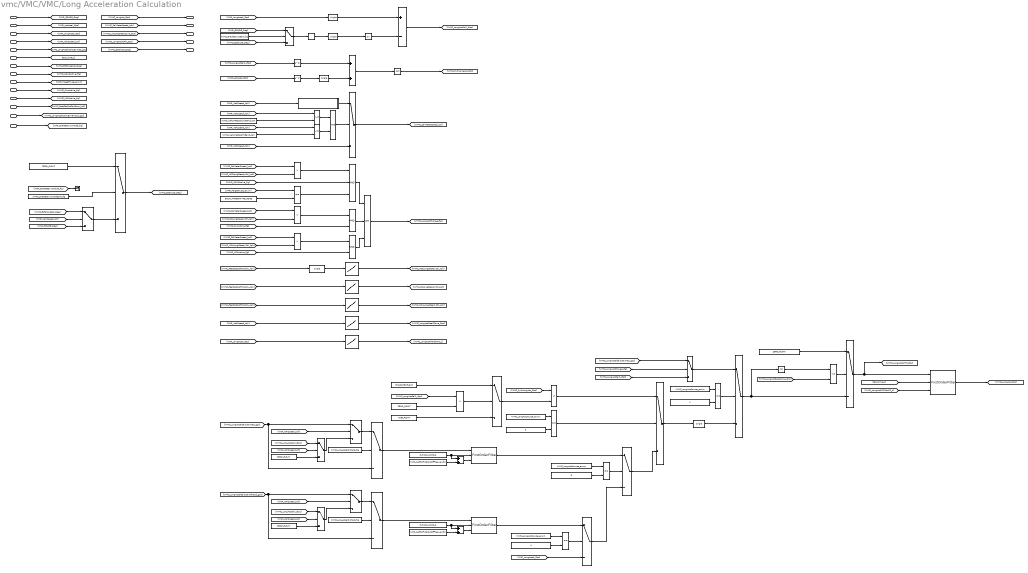
== system vmc/VMC/VMC/Long Acceleration Calculation ==
  VINP_GRADE_Deg : Inport
  VINP_LatAccel_Gps : Inport  Port=2
  VINP_LongAccel_Gps : Inport  Port=3
  VINP_VehSpeed_kph : Inport  Port=4
  VVMC_LongAccelCalcuByWSS_gps : Inport  Port=5
  task_time_s : Inport  Port=6
  VVMC_EstSlopeCal_Deg : Inport  Port=7
  VVMC_ADASActive_flg : Inport  Port=8
  VINP_TargetType_enum : Inport  Port=9
  VVMC_CruzActive_flg : Inport  Port=10
  VVMC_MSAActive_flg : Inport  Port=11
  VVMC_FeatSetSpdForCalcu_kph : Inport  Port=12
  VVMC_LongAccelCalcuByVehSpd_gps : Inport  Port=13
  VINP_DIDGetDynoMode_flg : Inport  Port=14
  AND : Logic  Inputs=3  AllPortsSameDT=off  OutDataTypeStr=boolean
  AND1 : Logic  AllPortsSameDT=off  OutDataTypeStr=boolean
  AND2 : Logic  AllPortsSameDT=off  OutDataTypeStr=boolean
  AND3 : Logic  AllPortsSameDT=off  OutDataTypeStr=boolean
  Abs : Abs
  Add1 : Sum
  Add2 : Sum  Inputs=+-
  Add3 : Sum
  Add9 : Sum
  Cast To Single{,1..2,4} (4 alike) : DataTypeConversion  OutDataTypeStr=single
  Constant : Constant  Value=KVMC_GradeSourceSW_flg
  Constant{1,7,16..17,22} (5 alike) : Constant  Value=ZERO_FLOAT
  Constant{5,10,12,14} (4 alike) : Constant  Value=KVMC_LongAccSource_enum
  Constant11 : Constant  Value=2  OutDataTypeStr=uint8
  Constant13 : Constant  OutDataTypeStr=uint8
  Constant15 : Constant  Value=4  OutDataTypeStr=uint8
  Constant18 : Constant  Value=KVMC_AccBWFilterCutOffFreq_raw32
  Constant19 : Constant  Value=KVMC_DIDGetDynoModeSW_flg
  Constant2 : Constant  Value=KVMC_Veh2MetSpdLowBand_kph
  Constant20 : Constant  Value=KVMC_LongAccelSWSpd_flg
  Constant21 : Constant  Value=C_TASK_10MS_S
  Constant27 : Constant  Value=KVMC_AccBWFilterCutOffFreq_raw32
  Constant29 : Constant  Value=C_TASK_10MS_S
  Constant3 : Constant  Value=KVMC_Veh2MetSpdHiBand_kph
  Constant30 : Constant  Value=KVMC_LongAccelSWSpd_flg
  Constant4 : Constant  Value=ENUM_TARGETTYPE_NONE
  Constant6 : Constant  Value=3  OutDataTypeStr=uint8
  Constant8 : Constant  Value=MINUSONE_FLOAT
  Constant9 : Constant  Value=ONE_FLOAT
  Data Type Conversion : DataTypeConversion  OutDataTypeStr=single
  Degrees to Radians1 : simulink_extras/Transformations/Degrees to Radians
  Equal{1..4} (4 alike) : RelationalOperator  Operator===  OutDataTypeStr=boolean  RndMeth=Simplest
  FirstOrderFilter : hcu_lib/Basic_Blocks/FirstOrderFilter
  FirstOrderFilter5 : hcu_lib/Basic_Blocks/FirstOrderFilter
  FirstOrderFilter8 : hcu_lib/Basic_Blocks/FirstOrderFilter
  MVMC_ACCLongSteadyCtrl_Y_kph : Lookup_n-D  NumberOfTableDimensions=1  BreakpointsForDimension1=AVMC_ACCLongSteadyCtrl_X_kph  Table=MVMC_ACCLongSteadyCtrl_Y_kph  ExtrapMethod=Clip  InternalRulePriority=Speed  RndMeth=Simplest  InputSameDT=on
  MVMC_CCLongSteadyCtrl_Y_kph : Lookup_n-D  NumberOfTableDimensions=1  BreakpointsForDimension1=AVMC_CCLongSteadyCtrl_X_kph  Table=MVMC_CCLongSteadyCtrl_Y_kph  ExtrapMethod=Clip  InternalRulePriority=Speed  RndMeth=Simplest  InputSameDT=on
  MVMC_LongAccDeadZone_Y_Gps : Lookup_n-D  NumberOfTableDimensions=1  BreakpointsForDimension1=AVMC_LongAccDeadZone_X_kph  Table=MVMC_LongAccDeadZone_Y_Gps  InternalRulePriority=Speed  RndMeth=Simplest  InputSameDT=on
  MVMC_LongAccFiltTsforP2_Y_c : Lookup_n-D  NumberOfTableDimensions=1  BreakpointsForDimension1=AVMC_LongAccFiltTsforP2_X_Gps  Table=MVMC_LongAccFiltTsforP2_Y_c  InternalRulePriority=Speed  RndMeth=Simplest  InputSameDT=on
  MVMC_MSALongSteadyCtrl_Y_kph : Lookup_n-D  NumberOfTableDimensions=1  BreakpointsForDimension1=AVMC_MSALongSteadyCtrl_X_kph  Table=MVMC_MSALongSteadyCtrl_Y_kph  ExtrapMethod=Clip  InternalRulePriority=Speed  RndMeth=Simplest  InputSameDT=on
  Math Function3 : Math  Operator=square  SaturateOnIntegerOverflow=on
  Math Function4 : Math  Operator=square  SaturateOnIntegerOverflow=on
  OR : Logic  Operator=OR  Inputs=3  AllPortsSameDT=off  OutDataTypeStr=boolean
  Product1 : Product
  Relational Operator1 : RelationalOperator  Operator=<  OutDataTypeStr=boolean  RndMeth=Simplest
  Relational Operator2 : RelationalOperator  Operator=<=  OutDataTypeStr=boolean  RndMeth=Simplest
  Relational Operator3 : RelationalOperator  Operator=>  OutDataTypeStr=boolean  RndMeth=Simplest
  Relational Operator4 : RelationalOperator  Operator===  OutDataTypeStr=boolean  RndMeth=Simplest
  Relational Operator5 : RelationalOperator  OutDataTypeStr=boolean  RndMeth=Simplest
  Relational Operator6 : RelationalOperator  Operator=<=  OutDataTypeStr=boolean  RndMeth=Simplest
  Relational Operator7 : RelationalOperator  Operator=>  OutDataTypeStr=boolean  RndMeth=Simplest
  Relational Operator8 : RelationalOperator  Operator=>  OutDataTypeStr=boolean  RndMeth=Simplest
  Sin1 : Trigonometry
  Square Root1 : Sqrt  SaturateOnIntegerOverflow=on
  Switch{,1..10,13..14,16} (14 alike) : Switch  Criteria=u2 > Threshold
  Switch11 : Switch  Criteria=u2 > Threshold  Threshold=KVMC_LongAccelSWSpd_kph
  Switch12 : Switch  Criteria=u2 > Threshold  Threshold=KVMC_LongAccelSWSpd_kph
  Switch15 : Switch  Criteria=u2 > Threshold  Threshold=KVMC_LongAccelSWSpd_kph
  Terminator : Terminator
  Vehicle to Meter Speed : Subsystem
  VVMC_LongAcc_Gps : Outport
  VVMC_CalMeterSpeed_kph : Outport  Port=2
  VVMC_LongAccDeadZone_Gps : Outport  Port=3
  VVMC_LongAccNoFilt_Gps : Outport  Port=4
  VVMC_EstSlope_Deg : Outport  Port=5
  wires:
  Switch5/1 -> Switch1/3, Abs/1
  Constant1/1 -> Switch1/1
  [VVMC_LongAccDeadZone_Gps] -> Relational Operator2/2
  Abs/1 -> Relational Operator2/1
  Relational Operator2/1 -> Switch1/2
  [VINP_VehSpeed_kph] -> MVMC_LongAccDeadZone_Y_Gps/1
  MVMC_LongAccDeadZone_Y_Gps/1 -> [VVMC_LongAccDeadZone_Gps]  "VVMC_LongAccDeadZone_Gps"
  VINP_VehSpeed_kph/1 -> [VINP_VehSpeed_kph]
  Cast To Single2/1 -> Switch5/3
  Relational Operator1/1 -> Switch3/2  "VVMC_LongAccNeg_flg"
  Constant7/1 -> Relational Operator1/2
  Switch6/1 -> Switch5/1  "VVMC_ActLongAccSource1_Gps"
  [VVMC_PythLongAcc_Gps] -> Product1/1
  Constant9/1 -> Switch3/3
  Switch4/1 -> Cast To Single2/1
  Switch3/1 -> Product1/2
  Equal3/1 -> Switch5/2
  [VVMC_LongAccCal1_Gps] -> Relational Operator1/1
  Constant10/1 -> Equal2/1
  Equal2/1 -> Switch4/2
  Product1/1 -> Switch4/1  "VVMC_LongAccCal2_Gps"
  Constant11/1 -> Equal2/2
  Constant8/1 -> Switch3/1
  Constant13/1 -> Equal3/2
  Constant12/1 -> Equal3/1
  Cast To Single4/1 -> Add3/2
  Square Root1/1 -> [VVMC_PythLongAcc_Gps]  "VVMC_PythLongAcc_Gps"
  [VVMC_LongAccCal1_Gps] -> Math Function4/1
  Math Function3/1 -> Cast To Single4/1
  Math Function4/1 -> Add3/1
  Add3/1 -> Square Root1/1
  [VINP_LatAccel_Gps] -> Math Function3/1
  Degrees to Radians1/1 -> Cast To Single/1
  Cast To Single1/1 -> Add2/1
  [VINP_GRADE_Deg] -> Switch/1
  Cast To Single/1 -> Sin1/1  "VVMC_GRADE_rad"
  Sin1/1 -> Add2/2  "VVMC_SINEGRADE_Gps"
  Add2/1 -> [VVMC_LongAccCal1_Gps]  "VVMC_LongAccCal1_Gps"
  [VINP_LongAccel_Gps] -> Cast To Single1/1
  VINP_GRADE_Deg/1 -> [VINP_GRADE_Deg]
  VINP_LatAccel_Gps/1 -> [VINP_LatAccel_Gps]
  VINP_LongAccel_Gps/1 -> [VINP_LongAccel_Gps]
  [VVMC_LongAcc_Gps] -> VVMC_LongAcc_Gps/1
  Constant5/1 -> Equal1/1
  [VINP_LongAccel_Gps] -> Switch8/3
  Constant6/1 -> Equal1/2
  Equal1/1 -> Switch2/2
  Switch2/1 -> Switch4/3
  VVMC_LongAccelCalcuByWSS_gps/1 -> [VVMC_LongAccelCalcuByWSS_gps]
  FirstOrderFilter/1 -> [VVMC_LongAcc_Gps]  "VVMC_LongAcc_Gps"
  MVMC_LongAccFiltTsforP2_Y_c/1 -> [VVMC_LongAccFiltTsforP2_c]  "VVMC_LongAccFiltTsforP2_c"
  [VINP_LongAccel_Gps] -> MVMC_LongAccFiltTsforP2_Y_c/1
  task_time_s/1 -> [task_time_s]
  Switch/1 -> Degrees to Radians1/1
  Constant/1 -> Switch/2
  [VVMC_EstSlope_Deg] -> Switch/3
  VVMC_EstSlopeCal_Deg/1 -> [VVMC_EstSlopeCal_Deg]
  Constant3/1 -> Relational Operator6/2
  Relational Operator6/1 -> AND2/2
  [VINP_VehSpeed_kph] -> Switch7/3
  Vehicle to Meter Speed/1(OutputSpeed) -> Switch7/1
  Relational Operator5/1 -> AND2/1
  [VINP_VehSpeed_kph] -> Relational Operator6/1
  [VINP_VehSpeed_kph] -> Vehicle to Meter Speed/1(InputSpeed)
  AND2/1 -> Switch7/2
  Switch7/1 -> [VVMC_CalMeterSpeed_kph]  "VVMC_CalMeterSpeed_kph"
  Constant2/1 -> Relational Operator5/2
  [VINP_VehSpeed_kph] -> Relational Operator5/1
  Constant4/1 -> Relational Operator4/2
  [VVMC_CruzActive_flg] -> AND1/2
  [VVMC_MSALongSteadyCtrl_kph] -> Relational Operator8/2
  [VVMC_CalMeterSpeed_kph] -> Relational Operator8/1
  Relational Operator8/1 -> AND3/1
  [VVMC_MSAActive_flg] -> AND3/2
  AND1/1 -> OR/2
  AND3/1 -> OR/3
  [VVMC_CCLongSteadyCtrl_kph] -> Relational Operator7/2
  [VVMC_CalMeterSpeed_kph] -> Relational Operator7/1
  Relational Operator7/1 -> AND1/1
  Relational Operator4/1 -> AND/3
  AND/1 -> OR/1
  Relational Operator3/1 -> AND/1
  [VINP_TargetType_enum] -> Relational Operator4/1
  [VVMC_CalMeterSpeed_kph] -> Relational Operator3/1
  [VVMC_ACCLongSteadyCtrl_kph] -> Relational Operator3/2
  OR/1 -> [VVMC_LongAccChange_flg]  "VVMC_LongAccChange_flg"
  [VVMC_ADASActive_flg] -> AND/2
  [VVMC_FeatSetSpdForCalcu_kph] -> MVMC_MSALongSteadyCtrl_Y_kph/1
  Data Type Conversion/1 -> MVMC_ACCLongSteadyCtrl_Y_kph/1
  MVMC_CCLongSteadyCtrl_Y_kph/1 -> [VVMC_CCLongSteadyCtrl_kph]  "VVMC_CCLongSteadyCtrl_kph"
  MVMC_MSALongSteadyCtrl_Y_kph/1 -> [VVMC_MSALongSteadyCtrl_kph]  "VVMC_MSALongSteadyCtrl_kph"
  MVMC_ACCLongSteadyCtrl_Y_kph/1 -> [VVMC_ACCLongSteadyCtrl_kph]  "VVMC_ACCLongSteadyCtrl_kph"
  [VVMC_FeatSetSpdForCalcu_kph] -> Data Type Conversion/1
  [VVMC_FeatSetSpdForCalcu_kph] -> MVMC_CCLongSteadyCtrl_Y_kph/1
  [VVMC_LongAccFiltTsforP2_c] -> FirstOrderFilter/3
  [task_time_s] -> FirstOrderFilter/2
  Switch1/1 -> FirstOrderFilter/1, [VVMC_LongAccNoFilt_Gps]
  [VVMC_LongAccCal1_Gps] -> Switch6/3
  [VVMC_LongAccelCalcuByWSS_gps] -> Switch6/1
  [VVMC_LongAccChange_flg] -> Switch6/2
  [VVMC_CalMeterSpeed_kph] -> VVMC_CalMeterSpeed_kph/1
  VVMC_FeatSetSpdForCalcu_kph/1 -> [VVMC_FeatSetSpdForCalcu_kph]
  VVMC_MSAActive_flg/1 -> [VVMC_MSAActive_flg]
  VVMC_CruzActive_flg/1 -> [VVMC_CruzActive_flg]
  VINP_TargetType_enum/1 -> [VINP_TargetType_enum]
  VVMC_ADASActive_flg/1 -> [VVMC_ADASActive_flg]
  VVMC_LongAccelCalcuByVehSpd_gps/1 -> [VVMC_LongAccelCalcuByVehSpd_gps]
  Equal4/1 -> Switch8/2
  Constant15/1 -> Equal4/2
  Constant14/1 -> Equal4/1
  Switch8/1 -> Switch2/3
  Switch12/1 -> Switch9/1
  Switch9/1 -> FirstOrderFilter5/1
  Constant21/1 -> FirstOrderFilter5/2, Add1/1
  Constant29/1 -> Add9/1, FirstOrderFilter8/2
  [VINP_VehSpeed_kph] -> Switch11/2
  Add9/1 -> FirstOrderFilter8/3
  Constant30/1 -> Switch10/2
  Add1/1 -> FirstOrderFilter5/3
  Switch11/1 -> Switch10/1
  [VVMC_LongAccelCalcuByVehSpd_gps] -> Switch11/1, Switch10/3
  Switch10/1 -> FirstOrderFilter8/1
  Constant20/1 -> Switch9/2
  Constant27/1 -> Add9/2
  [VINP_VehSpeed_kph] -> Switch12/2
  [VVMC_LongAccelCalcuByWSS_gps] -> Switch12/1, Switch9/3
  Constant18/1 -> Add1/2
  Switch13/1 -> Switch12/3
  FirstOrderFilter8/1 -> Switch8/1  "VVMC_LongAccelCalcuByVehSpd_gps"
  FirstOrderFilter5/1 -> Switch2/1  "VVMC_LongAccelCalcuByWSS_gps"
  [VVMC_LongAccDeadZone_Gps] -> VVMC_LongAccDeadZone_Gps/1
  [VINP_VehSpeed_kph] -> Switch13/2
  [VVMC_LongAccCal1_Gps] -> Switch13/1
  Constant16/1 -> Switch13/3
  Constant17/1 -> Switch14/3
  [VVMC_LongAccCal1_Gps] -> Switch14/1
  [VINP_VehSpeed_kph] -> Switch14/2
  Switch14/1 -> Switch11/3
  [VVMC_LongAccNoFilt_Gps] -> VVMC_LongAccNoFilt_Gps/1
  [VINP_VehSpeed_kph] -> Switch15/2
  [VINP_GRADE_Deg] -> Switch15/3
  [VVMC_EstSlopeCal_Deg] -> Switch15/1
  Switch16/1 -> [VVMC_EstSlope_Deg]  "VVMC_EstSlope_Deg"
  [VVMC_EstSlope_Deg] -> VVMC_EstSlope_Deg/1
  Switch15/1 -> Switch16/3
  Constant22/1 -> Switch16/1
  Constant19/1 -> Switch16/2
  VINP_DIDGetDynoMode_flg/1 -> [VINP_DIDGetDynoMode_flg]
  [VINP_DIDGetDynoMode_flg] -> Terminator/1

== system vmc/VMC/VMC/MSA function ==
  VTQD_ExternalTqAllow_flg : Inport
  VTQD_DriverWhlTqDem_Nm : Inport  Port=2
  <VINP_ZoneSpdCtrlMode_enum> : Inport  Port=3
  VINP_SWCCANCELSta_flg : Inport  Port=4
  VINP_VehSpeed_kph : Inport  Port=5
  VVMC_LongAcc_Gps : Inport  Port=6
  VVMC_FeatSetSpdForCalcu_kph : Inport  Port=7
  VVMC_FeatArbitrFinal_enum : Inport  Port=8
  VINP_SWCResUpSta_flg : Inport  Port=9
  VINP_SWCSetdownSta_flg : Inport  Port=10
  VVMC_MeterIndSpeedForCalcu_kph : Inport  Port=11
  VTQD_LowIdleAccPedal_flg : Inport  Port=12
  VDHP_ActAPSPosn_pct : Inport  Port=13
  task_time_s : Inport  Port=14
  VVMC_ActACCRequiredAccel_mps2 : Inport  Port=15
  VTQR_FrTMTqReq_Nm : Inport  Port=16
  VTQR_RrTMTqReq_Nm : Inport  Port=17
  VVMC_TotalAvailBrkRgnTq_Nm : Inport  Port=18
  VINP_HoodSW_flg : Inport  Port=19
  VTQD_GearActualPosn_enum : Inport  Port=20
  Add : Sum  Inputs=+-
  Anti-Speed Limitation : Subsystem
  Constant : Constant  Value=TRUE
  Constant1 : Constant  Value=KVMC_CCMSASpdWar_kph
  Constant2 : Constant  Value=KVMC_AntiSpdLim_kph
  Constant3 : Constant  Value=ENUM_ADASMSASTA_ANTILIMIT
  Constant4 : Constant  Value=KVMC_AntiSpdLim_kph
  Constant5 : Constant  Value=KVMC_AntiSpdLim_kph
  Data Type Conversion : DataTypeConversion  OutDataTypeStr=single
  MSAActivationHandshake : Subsystem
  MSADemandTorqueCalculation : Subsystem
  MSATorqueSourceDetermination : Subsystem
  Relational Operator : RelationalOperator  OutDataTypeStr=boolean  RndMeth=Simplest
  Switch{,1..4} (5 alike) : Switch  Criteria=u2 > Threshold
  Unit Delay : UnitDelay  SampleTime=-1  HasFrameUpgradeWarning=on
  VVMC_MSACtrlSta_enum : Outport
  VVMC_MSAWhlTqReq_Nm : Outport  Port=2
  VVMC_MSASpdWar_flg : Outport  Port=3
  VVMC_MSAActive_flg : Outport  Port=4
  VVMC_MSAWhlTqActive_flg : Outport  Port=5
  VVMC_AntiSpdLimEn_flg : Outport  Port=6
  wires:
  [VVMC_MSAWhlTqActive_flg] -> VVMC_MSAWhlTqActive_flg/1
  MSATorqueSourceDetermination/3(VVMC_MSAWhlTqActive_flg) -> [VVMC_MSAWhlTqActive_flg]
  [VVMC_MSAActive_flg] -> MSATorqueSourceDetermination/9(VVMC_MSAActive_flg)
  Unit Delay/1 -> MSAActivationHandshake/9(VVMC_MSAOvrdAllow_flg)
  [VVMC_MSAOvrdAllow_flg] -> Unit Delay/1
  [VVMC_MeterIndSpeedForCalcu_kph] -> MSATorqueSourceDetermination/8(VVMC_MeterIndSpeedForCalcu_kph)
  [VTQD_LowIdleAccPedal_flg] -> MSADemandTorqueCalculation/12(VTQD_LowIdleAccPedal_flg)
  [task_time_s] -> MSADemandTorqueCalculation/11(task_time_s)
  MSATorqueSourceDetermination/2(VVMC_MSAOvrdAllow_flg) -> [VVMC_MSAOvrdAllow_flg]
  [VVMC_MSAOvrdAllow_flg] -> MSADemandTorqueCalculation/10(VVMC_MSAPedalOvrd_flg)
  [VTQR_RrTMTqReq_Nm] -> MSADemandTorqueCalculation/9(VTQR_RrTMTqReq_Nm)
  [VTQR_FrTMTqReq_Nm] -> MSADemandTorqueCalculation/8(VTQR_FrTMTqReq_Nm)
  VTQR_RrTMTqReq_Nm/1 -> [VTQR_RrTMTqReq_Nm]
  VTQR_FrTMTqReq_Nm/1 -> [VTQR_FrTMTqReq_Nm]
  [VVMC_ActACCRequiredAccel_mps2] -> MSADemandTorqueCalculation/7(VVMC_ActACCRequiredAccel_mps2)
  VVMC_ActACCRequiredAccel_mps2/1 -> [VVMC_ActACCRequiredAccel_mps2]
  Switch4/1 -> MSATorqueSourceDetermination/7(VVMC_FeatSetSpdForCalcu_kph)
  [task_time_s] -> MSATorqueSourceDetermination/6(task_time_s)
  task_time_s/1 -> [task_time_s]
  [VINP_VehSpeed_kph] -> MSATorqueSourceDetermination/5(VINP_VehSpeed_kph)
  [VDHP_ActAPSPosn_pct] -> MSATorqueSourceDetermination/4(VDHP_ActAPSPosn_pct)
  [VTQD_LowIdleAccPedal_flg] -> MSATorqueSourceDetermination/3(VTQD_LowIdleAccPedal_flg)
  VTQD_LowIdleAccPedal_flg/1 -> [VTQD_LowIdleAccPedal_flg]
  VDHP_ActAPSPosn_pct/1 -> [VDHP_ActAPSPosn_pct]
  [VVMC_MeterIndSpeedForCalcu_kph] -> MSADemandTorqueCalculation/6(VVMC_MeterIndSpeedForCalcu_kph)
  VVMC_MeterIndSpeedForCalcu_kph/1 -> [VVMC_MeterIndSpeedForCalcu_kph]
  [VVMC_LongAcc_Gps] -> MSADemandTorqueCalculation/5(VVMC_LongAcc_Gps)
  VVMC_LongAcc_Gps/1 -> [VVMC_LongAcc_Gps]
  [VVMC_MeterIndSpeedForCalcu_kph] -> MSAActivationHandshake/4(VVMC_MeterIndSpeedForCalcu_kph)
  [VINP_VehSpeed_kph] -> MSADemandTorqueCalculation/2(VINP_VehSpeed_kph)
  VINP_VehSpeed_kph/1 -> [VINP_VehSpeed_kph]
  [VVMC_MSAActive_flg] -> VVMC_MSAActive_flg/1
  Data Type Conversion/1 -> [VVMC_FeatSetSpdForCalcu_kph]  "VVMC_FeatSetSpdForCalcu_kph"
  [VVMC_MSAWhlTqReq_Nm] -> VVMC_MSAWhlTqReq_Nm/1
  [VVMC_MSASpdWar_flg] -> VVMC_MSASpdWar_flg/1
  [VVMC_MSACtrlSta_enum] -> VVMC_MSACtrlSta_enum/1
  VTQD_DriverWhlTqDem_Nm/1 -> [VTQD_DriverWhlTqDem_Nm]
  VINP_SWCCANCELSta_flg/1 -> [VINP_SWCCANCELSta_flg]
  VVMC_FeatSetSpdForCalcu_kph/1 -> Data Type Conversion/1
  VTQD_ExternalTqAllow_flg/1 -> [VTQD_ExternalTqAllow_flg]
  VVMC_FeatArbitrFinal_enum/1 -> [VVMC_FeatArbitrFinal_enum]
  [VTQD_DriverWhlTqDem_Nm] -> MSATorqueSourceDetermination/2(VTQD_DriverWhlTqDem_Nm)
  [VTQD_DriverWhlTqDem_Nm] -> MSADemandTorqueCalculation/4(VTQD_DriverWhlTqDem_Nm)
  [VVMC_FeatSetSpdForCalcu_kph] -> Switch3/3
  [VINP_SWCCANCELSta_flg] -> MSAActivationHandshake/6(VINP_SWCCANCELSta_flg)
  [VVMC_FeatSetSpdForCalcu_kph] -> MSAActivationHandshake/5(VVMC_FeatSetSpdForCalcu_kph)
  [VTQD_ExternalTqAllow_flg] -> MSAActivationHandshake/3(VTQD_ExternalTqAllow_flg)
  [VVMC_FeatArbitrFinal_enum] -> MSAActivationHandshake/2(VVMC_FeatArbitrFinal_enum)
  MSATorqueSourceDetermination/1(VVMC_MSAWhlTqReq_Nm) -> [VVMC_MSAWhlTqReq_Nm]
  [VVMC_MSAWhlTqCal_Nm] -> MSATorqueSourceDetermination/1(VVMC_MSAWhlTqCal_Nm)
  MSADemandTorqueCalculation/1(VVMC_MSAWhlTqCal_Nm) -> [VVMC_MSAWhlTqCal_Nm]
  [VVMC_MSAActive_flg] -> MSADemandTorqueCalculation/3(VVMC_MSAActive_flg)
  Switch/1 -> [VVMC_MSAActive_flg]  "VVMC_MSAActive_flg"
  Switch1/1 -> [VVMC_MSASpdWar_flg]  "VVMC_MSASpdWar_flg"
  Switch2/1 -> [VVMC_MSACtrlSta_enum]  "VVMC_MSACtrlSta_enum"
  <VINP_ZoneSpdCtrlMode_enum>/1 -> [VINP_ZoneSpdCtrlMode_enum]
  [VINP_ZoneSpdCtrlMode_enum] -> MSAActivationHandshake/1(VINP_ZoneSpdCtrlMode_enum)
  VINP_SWCSetdownSta_flg/1 -> [VINP_SWCSetdownSta_flg]
  VINP_SWCResUpSta_flg/1 -> [VINP_SWCResUpSta_flg]
  [VINP_SWCResUpSta_flg] -> MSAActivationHandshake/7(VINP_SWCResUpSta_flg)  "VINP_SWCResUpSta_flg"
  [VINP_SWCSetdownSta_flg] -> MSAActivationHandshake/8(VINP_SWCSetdownSta_flg)  "VINP_SWCSetdownSta_flg"
  [VINP_SWCResUpSta_flg] -> MSADemandTorqueCalculation/13(VINP_SWCResUpSta_flg)  "VINP_SWCResUpSta_flg"
  [VINP_SWCResUpSta_flg] -> MSATorqueSourceDetermination/10(VINP_SWCResUpSta_flg)  "VINP_SWCResUpSta_flg"
  VVMC_TotalAvailBrkRgnTq_Nm/1 -> [VVMC_TotalAvailBrkRgnTq_Nm]
  [VVMC_TotalAvailBrkRgnTq_Nm] -> MSADemandTorqueCalculation/14(VVMC_TotalAvailBrkRgnTq_Nm)
  VINP_HoodSW_flg/1 -> [VINP_HoodSW_flg]
  Anti-Speed Limitation/1(VVMC_AntiSpdLimEn_flg) -> [VVMC_AntiSpdLimEn_flg]
  [VTQD_GearActualPosn_enum] -> Anti-Speed Limitation/2(VTQD_GearActualPosn_enum)
  [VINP_HoodSW_flg] -> Anti-Speed Limitation/1(VINP_HoodSW_flg)
  VTQD_GearActualPosn_enum/1 -> [VTQD_GearActualPosn_enum]
  [VVMC_AntiSpdLimEn_flg] -> Switch/2
  MSAActivationHandshake/3(VVMC_MSAActive_flg) -> Switch/3
  Constant/1 -> Switch/1
  Relational Operator/1 -> Switch1/1
  [VVMC_AntiSpdLimEn_flg] -> Switch1/2
  MSAActivationHandshake/2(VVMC_MSASpdWar_flg) -> Switch1/3
  [VVMC_MeterIndSpeedForCalcu_kph] -> Add/1
  Constant2/1 -> Add/2
  Add/1 -> Relational Operator/1
  Constant1/1 -> Relational Operator/2
  Constant3/1 -> Switch2/1
  [VVMC_AntiSpdLimEn_flg] -> Switch2/2
  MSAActivationHandshake/1(VVMC_MSACtrlSta_enum) -> Switch2/3
  [VVMC_AntiSpdLimEn_flg] -> Switch3/2
  Switch3/1 -> MSADemandTorqueCalculation/1(VVMC_FeatSetSpdForCalcu_kph)
  Constant4/1 -> Switch3/1
  Constant5/1 -> Switch4/1
  [VVMC_AntiSpdLimEn_flg] -> Switch4/2
  [VVMC_FeatSetSpdForCalcu_kph] -> Switch4/3
  [VVMC_AntiSpdLimEn_flg] -> VVMC_AntiSpdLimEn_flg/1
  [VVMC_AntiSpdLimEn_flg] -> MSATorqueSourceDetermination/11(VVMC_AntiSpdLimEn_flg)
